simulink model "single_track"  (R2020a)
settings: Solver=ode23tb  StartTime=0  MaxStep=0.1  RelTol=1e-3  AbsTol=1e-6  EnableMultiTasking=on
values from neighbouring files (symbols this model uses):
  kp = 500    [main.m]    (also in main_test.m)
  Ts = STEP_STEER.time(2)-STEP_STEER.time(1)    [main.m]    (also in main_test.m)
  U0 = 95.0/3.6    (= 26.3888888889)    [main.m]    (also in main_test.m = mean(STEP_STEER.long_vel); parametric_simulations.m = u0)
settings Model: Creator=francescobiral  LastModifiedBy=Pasquale Romano
settings DataIOCC: InitialState=init_states1  LoadInitialState=on  SaveFormat=Array  SaveState=on  ReturnWorkspaceOutputs=off
settings OptimizationCC: LifeSpan=inf
settings DebuggingCC: UnderspecifiedInitializationDetection=Classic  MergeDetectMultiDrivingBlocksExec=none  SolverPrmCheckMsg=warning  StateNameClashWarn=warning  SFUnexpectedBacktrackingDiag=warning  SFNoUnconditionalDefaultTransitionDiag=warning  SFExecutionAtInitializationDiag=none  ArithmeticOperatorsInVariantConditions=warning
settings HardwareCC: ProdBitPerPointer=32  ProdBitPerSizeT=32  ProdBitPerPtrDiffT=32  ProdLargestAtomicFloat=None  ProdIntDivRoundTo=Undefined  ProdEndianess=Unspecified  ProdWordSize=32  ProdHWDeviceType=32-bit Generic
settings ModelReferenceCC: PropagateSignalLabelsOutOfModel=off
settings SFSimCC: SimUseLocalCustomCode=off  CustomCodeUndefinedFunction=UseInterfaceOnly
settings RTWCC: RTWUseLocalCustomCode=off
settings CodeAppCC: StateflowObjectComments=on
settings GRTTargetCC: TargetLangStandard=C89/C90 (ANSI)
settings ConfigComp: CovMetricSettings=dw  CovHtmlReporting=on  CovSaveCumulativeToWorkspaceVar=on  CovSaveSingleToWorkspaceVar=on  CovExternalEMLEnable=off

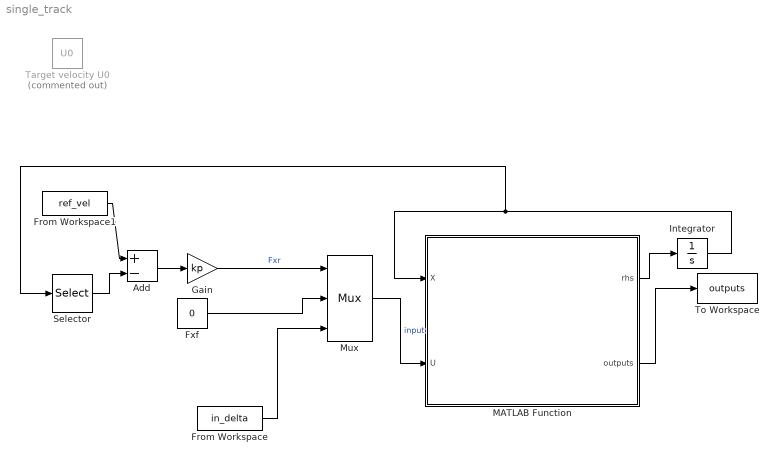
== system single_track ==
  Add : Sum  Inputs=+-
  From Workspace : FromWorkspace  VariableName=in_delta  SampleTime=Ts  OutputAfterFinalValue=Holding final value
  From Workspace1 : FromWorkspace  VariableName=ref_vel  SampleTime=Ts
  Fxf : Constant  Value=0
  Gain : Gain  Gain=kp
  Integrator : Integrator
  MATLAB Function : MATLAB Function  TreatAsAtomicUnit=on
  Mux : Mux  Inputs=3
      settings: DisplayOption=signals
  Selector : Selector  InputPortWidth=6  IndexOptions=Index vector (dialog)  Indices=[4]  OutputSizes=1
  Target velocity U0 : Constant  Commented=on  Value=U0
  To Workspace : ToWorkspace  VariableName=outputs  SampleTime=-1
  wires:
  MATLAB Function/1(rhs) -> Integrator/1
  Add/1 -> Gain/1
  Integrator/1 -> Selector/1, MATLAB Function/1(X)
  Selector/1 -> Add/2
  MATLAB Function/2(outputs) -> To Workspace/1
  Mux/1 -> MATLAB Function/2(U)  "input"
  From Workspace/1 -> Mux/3
  Fxf/1 -> Mux/2
  Gain/1 -> Mux/1  "Fxr"
  From Workspace1/1 -> Add/1

== matlab function single_track/MATLAB Function ==
  data: X input; U input; rhs output; data parameter; outputs output
function [rhs, outputs] = single_track_dynamics(X,U,data)
  
%   %extract data
  g     = data.gravity;
  M     = data.mass;
  Iz    = data.Iz;
  L__r  = data.Lr;
  L__f  = data.Lf;
  k__v  = data.kv;
  h     = data.h;
  %
  Byr = data.Byr;
  Cyr = data.Cyr;
  Dyr = data.Dyr;
  Eyr = data.Eyr;
  Kyr = data.Kyr;
  
  Byf = data.Byf;
  Cyf = data.Cyf;
  Dyf = data.Dyf;
  Eyf = data.Eyf;
  Kyf = data.Kyf;
  
  % initialization of vectors ---------------------------------------------
  rhs     = zeros(6,1);
  outputs = zeros(6,1);

  % calculate side slips (linear model) -----------------------------------
  alpha__r = -(-X(6) * L__r + X(5)) / X(4);
  alpha__f = U(3) - (X(6) * L__f + X(5)) / X(4);

 
  % calculate forces ------------------------------------------------------
  DN  = +(U(1)+U(2)-k__v*X(4)^2)*h/(L__r+L__f); %load transfer
  F__zr = M*g*L__f/(L__r+L__f)+DN;
  F__zf = M*g*L__r/(L__r+L__f)-DN;
  
  
  switch data.tyre_model
    case 1 % linear tyre model
   F__yr = Kyr*alpha__r*F__zr; %Kyr*alpha_r*Fzr;
   F__yf = Kyf*alpha__f*F__zf; %kyf*alpha_f*Fzf;
    case 2 % non-linear tyre model
  %phi_r = sqrt(1-(U(1)/(Fzr*Dyr))^2); % scaling factor for combined slip (rear)
  %phi_f = sqrt(1-(U(2)/(Fzf*Dyf))^2); % scaling factor for combined slip (front)
    F__yr = magic_formula(alpha__r,Byr,Cyr,Dyr,Eyr)*F__zr; %*phi_r
    F__yf = magic_formula(alpha__f,Byf,Cyf,Dyf,Eyf)*F__zf; %*phi_f 
    otherwise 
      error 'unknonw tyre model'
  end
  
  % vector of system output
  outputs(1) = F__zr;
  outputs(2) = F__zf;
  outputs(3) = alpha__r;
  outputs(4) = alpha__f;
  outputs(5) = F__yr;
  outputs(6) = F__yf;
  
  % calculate dx/dt rhs of ode system
  % (automatically generated)
  t1 = sin(X(3));
  t3 = cos(X(3));
  t11 = X(4) ^ 2;
  t15 = 0.1e1 / M;
  rhs(1) = -t1 * X(5) + t3 * X(4);
  rhs(2) = t1 * X(4) + t3 * X(5);
  rhs(3) = X(6);
  rhs(4) = t15 * (M * X(5) * X(6) - F__yf * U(3) - t11 * k__v + U(1) + U(2));
  rhs(5) = t15 * (-M * X(4) * X(6) + U(2) * U(3) + F__yf + F__yr);
  rhs(6) = (L__f * U(2) * U(3) + F__yf * L__f - F__yr * L__r) / Iz;

end
